simulink model "HeadAgent"  (Simulink 6.5)
settings: Solver=ode45  StartTime=0.0  StopTime=10.0  RelTol=1e-3
settings Model: Creator=suarezjl  LastModifiedBy=suarezjl
settings DataIOCC: SignalLoggingName=sigsOut
settings DebuggingCC: SolverPrmCheckMsg=none  MultiTaskDSMMsg=warning  MultiTaskCondExecSysMsg=none  StrictBusMsg=None
settings HardwareCC: TargetUnknown=on
settings RTWCC: IncludeERTFirstTime=on

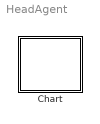
== system HeadAgent ==
  Chart : Stateflow chart

== stateflow chart Chart ==
  state Initialize
    \\Sally\RightReachDemo\HeadModule\HeadAgent\EyeMotionControl.Initial()
  state MainLoop
    \\Sally\RightReachDemo\HeadModule\HeadAgent\EyeMotionControl.HeadSample()
    \\Sally\RightReachDemo\HeadModule\HeadAgent\EyeMotionControl.DoProportionalTracking()
    \\Sally\RightReachDemo\HeadModule\HeadAgent\EyeMotionControl.WriteMotorPositions()
    \\Sally\RightReachDemo\HeadModule\HeadAgent\DepthEstimator.FindCartesianCoordinates()
  state Stop
    \\Sally\RightReachDemo\HeadModule\HeadAgent\EyeMotionControl.Initial()
  Initialize -> MainLoop : Always
  MainLoop -> MainLoop [order 1] : Always
  (default) -> Initialize : Start
  MainLoop -> Stop [order 2] : Signal="Stop"
